simulink model "Lab2_ball_beam"  (Simulink 9.2)
settings: Solver=ode45  StartTime=0.0  StopTime=40  MaxStep=0.001  RelTol=1e-3  AbsTol=1e-6
settings Model: Creator=Shaocheng  LastModifiedBy=buddyugwumba1
settings SolverCC: AutoScaleAbsTol=off
settings DataIOCC: LimitDataPoints=off  Refine=4
settings OptimizationCC: BlockReduction=off  BooleanDataType=off  ExpressionDepthLimit=2147483647  InitFltsAndDblsToZero=on
settings DebuggingCC: SaveWithParameterizedLinksMsg=none  SignalResolutionControl=TryResolveAllWithWarning  MultiTaskDSMMsg=warning  MultiTaskCondExecSysMsg=none
settings HardwareCC: TargetUnknown=on
settings GRTTargetCC: TargetFcnLib=ansi_tfl_tmw.mat

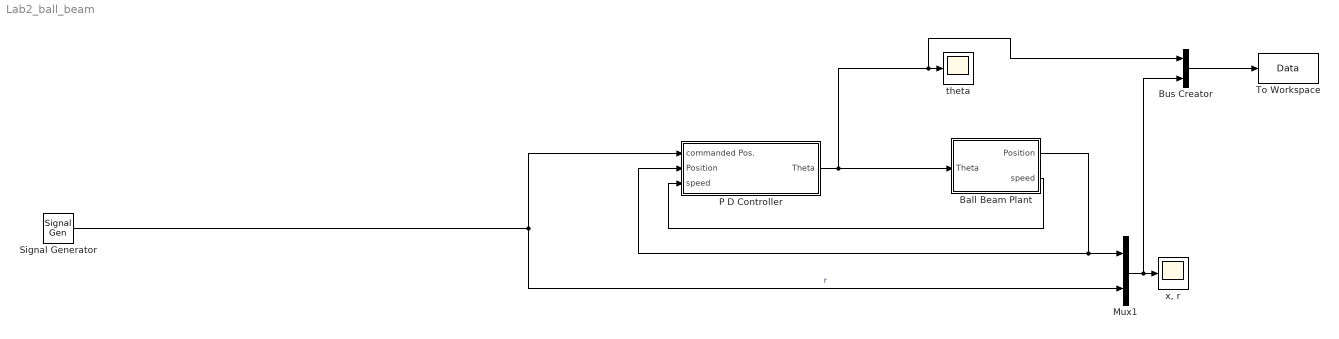
== system Lab2_ball_beam ==
  Ball Beam Plant : Subsystem
  Bus Creator : BusCreator  Inputs=2
  Mux1 : Mux  Inputs=2
  P D Controller : Subsystem
  Signal Generator : SignalGenerator  Amplitude=0.25  Units=rad/sec
  To Workspace : ToWorkspace  VariableName=Data  SaveFormat=Structure With Time  SampleTime=-1
  theta : Scope
  "x, r" : Scope
  wires:
  Mux1/1 -> Bus Creator/2, "x, r"/1
  P D Controller/1(Theta) -> Ball Beam Plant/1(Theta), Bus Creator/1, theta/1
  Ball Beam Plant/1(Position) -> Mux1/1, P D Controller/2(Position)
  Signal Generator/1 -> Mux1/2, P D Controller/1(commanded Pos.)  "r"
  Ball Beam Plant/2(speed) -> P D Controller/3(speed)
  Bus Creator/1 -> To Workspace/1

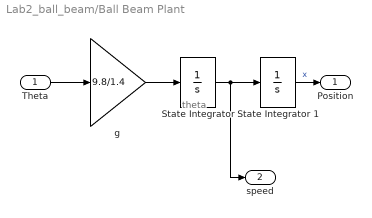
== system Lab2_ball_beam/Ball Beam Plant ==
  note: theta
  Theta : Inport
  State Integrator : Integrator  InitialCondition=0.1
  State Integrator 1 : Integrator
  g : Gain  Gain=9.8/1.4
  Position : Outport
  speed : Outport  Port=2
  wires:
  State Integrator/1 -> State Integrator 1/1, speed/1
  g/1 -> State Integrator/1
  Theta/1 -> g/1
  State Integrator 1/1 -> Position/1  "x"

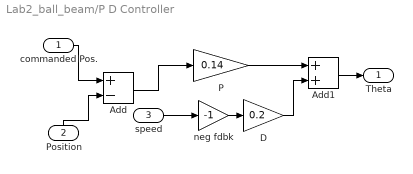
== system Lab2_ball_beam/P D Controller ==
  commanded Pos. : Inport
  Position : Inport  Port=2
  speed : Inport  Port=3
  Add : Sum  Inputs=+-
  Add1 : Sum
  D : Gain  Gain=0.2
  P : Gain  Gain=0.14
  neg fdbk : Gain  Gain=-1
  Theta : Outport
  wires:
  Add/1 -> P/1
  D/1 -> Add1/2
  P/1 -> Add1/1
  commanded Pos./1 -> Add/1
  Position/1 -> Add/2
  Add1/1 -> Theta/1
  speed/1 -> neg fdbk/1
  neg fdbk/1 -> D/1
